simulink model "generic_20231123_1032"  (R2022b)
settings: Solver=ode45  StartTime=0.0  StopTime=50  RelTol=1e-3  EnableMultiTasking=on
model workspace (MAT data in the model file):
  A = 1
  B = 1.19071237887
  kd = -9.99955278144
  ki = 0.00519416981022
  kp = 9.99999979837
undefined symbols (not defined in the file): brake_select, curvature, DiscIntNeverNeededParam, speed
libraries: CarMaker4SL x88, simulink x1, mpcadaslib x1
(part 2 of 4)

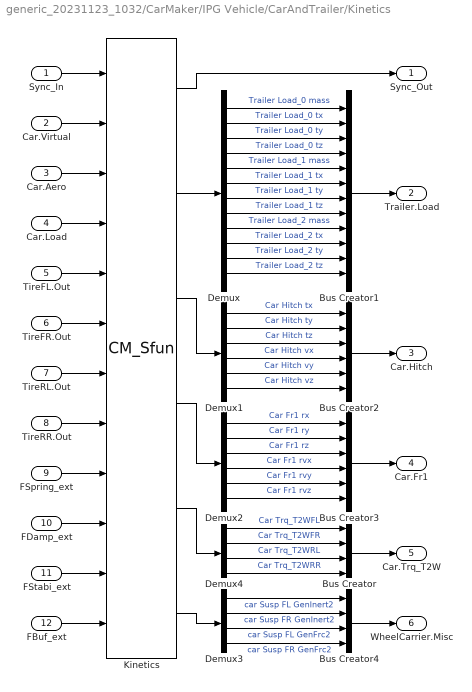
== system generic_20231123_1032/CarMaker/IPG Vehicle/CarAndTrailer/Kinetics ==
  Sync_In : Inport
  Car.Virtual : Inport  Port=2
  Car.Aero : Inport  Port=3
  Car.Load : Inport  Port=4
  TireFL.Out : Inport  Port=5
  TireFR.Out : Inport  Port=6
  TireRL.Out : Inport  Port=7
  TireRR.Out : Inport  Port=8
  FSpring_ext : Inport  Port=9
  FDamp_ext : Inport  Port=10
  FStabi_ext : Inport  Port=11
  FBuf_ext : Inport  Port=12
  Bus Creator : BusCreator  Inputs=4
  Bus Creator1 : BusCreator  Inputs=12
  Bus Creator2 : BusCreator  Inputs=6
  Bus Creator3 : BusCreator  Inputs=6
  Bus Creator4 : BusCreator  Inputs=4
  Demux : Demux  Outputs=12
      settings: DisplayOption=none
  Demux1 : Demux  Outputs=6
      settings: DisplayOption=none
  Demux2 : Demux  Outputs=6
      settings: DisplayOption=none
  Demux3 : Demux
      settings: DisplayOption=none
  Demux4 : Demux
      settings: DisplayOption=none
  Kinetics : S-Function  FunctionName=CM_Sfun  Parameters='Kinetics'  SFunctionDeploymentMode=off  EnableBusSupport=off
  Sync_Out : Outport  VectorParamsAs1DForOutWhenUnconnected=off
  Trailer.Load : Outport  Port=2  VectorParamsAs1DForOutWhenUnconnected=off
  Car.Hitch : Outport  Port=3  VectorParamsAs1DForOutWhenUnconnected=off
  Car.Fr1 : Outport  Port=4  VectorParamsAs1DForOutWhenUnconnected=off
  Car.Trq_T2W : Outport  Port=5  VectorParamsAs1DForOutWhenUnconnected=off
  WheelCarrier.Misc : Outport  Port=6  VectorParamsAs1DForOutWhenUnconnected=off
  wires:
  FBuf_ext/1 -> Kinetics/12
  Sync_In/1 -> Kinetics/1
  Kinetics/1 -> Sync_Out/1
  Car.Aero/1 -> Kinetics/3
  Car.Virtual/1 -> Kinetics/2
  Bus Creator1/1 -> Trailer.Load/1
  Demux/1 -> Bus Creator1/1  "Trailer Load_0 mass"
  Demux/2 -> Bus Creator1/2  "Trailer Load_0 tx"
  Demux/3 -> Bus Creator1/3  "Trailer Load_0 ty"
  Demux/4 -> Bus Creator1/4  "Trailer Load_0 tz"
  Kinetics/2 -> Demux/1
  Demux/5 -> Bus Creator1/5  "Trailer Load_1 mass"
  Demux/6 -> Bus Creator1/6  "Trailer Load_1 tx"
  Demux/7 -> Bus Creator1/7  "Trailer Load_1 ty"
  Demux/8 -> Bus Creator1/8  "Trailer Load_1 tz"
  Demux/9 -> Bus Creator1/9  "Trailer Load_2 mass"
  Demux/10 -> Bus Creator1/10  "Trailer Load_2 tx"
  Demux/11 -> Bus Creator1/11  "Trailer Load_2 ty"
  Demux/12 -> Bus Creator1/12  "Trailer Load_2 tz"
  Demux1/1 -> Bus Creator2/1  "Car Hitch tx"
  Demux1/2 -> Bus Creator2/2  "Car Hitch ty"
  Demux1/3 -> Bus Creator2/3  "Car Hitch tz"
  Demux1/4 -> Bus Creator2/4  "Car Hitch vx"
  Demux1/5 -> Bus Creator2/5  "Car Hitch vy"
  Demux1/6 -> Bus Creator2/6  "Car Hitch vz"
  Kinetics/3 -> Demux1/1
  Bus Creator2/1 -> Car.Hitch/1
  Demux2/1 -> Bus Creator3/1  "Car Fr1 rx"
  Demux2/2 -> Bus Creator3/2  "Car Fr1 ry"
  Demux2/3 -> Bus Creator3/3  "Car Fr1 rz"
  Demux2/4 -> Bus Creator3/4  "Car Fr1 rvx"
  Demux2/5 -> Bus Creator3/5  "Car Fr1 rvy"
  Demux2/6 -> Bus Creator3/6  "Car Fr1 rvz"
  Bus Creator3/1 -> Car.Fr1/1
  Kinetics/4 -> Demux2/1
  Car.Load/1 -> Kinetics/4
  Demux3/1 -> Bus Creator4/1  "car Susp FL GenInert2"
  Demux3/2 -> Bus Creator4/2  "car Susp FR GenInert2"
  Demux3/3 -> Bus Creator4/3  "car Susp FL GenFrc2"
  Demux3/4 -> Bus Creator4/4  "car Susp FR GenFrc2"
  Bus Creator4/1 -> WheelCarrier.Misc/1
  Bus Creator/1 -> Car.Trq_T2W/1
  Demux4/4 -> Bus Creator/4  "Car Trq_T2WRR"
  Demux4/3 -> Bus Creator/3  "Car Trq_T2WRL"
  Demux4/2 -> Bus Creator/2  "Car Trq_T2WFR"
  Demux4/1 -> Bus Creator/1  "Car Trq_T2WFL"
  TireFL.Out/1 -> Kinetics/5
  TireFR.Out/1 -> Kinetics/6
  TireRL.Out/1 -> Kinetics/7
  TireRR.Out/1 -> Kinetics/8
  FSpring_ext/1 -> Kinetics/9
  FDamp_ext/1 -> Kinetics/10
  FStabi_ext/1 -> Kinetics/11
  Kinetics/6 -> Demux3/1
  Kinetics/5 -> Demux4/1

== system generic_20231123_1032/CarMaker/IPG Vehicle/CarAndTrailer/Steering ==
  note: When replacing the entire steering system,
      | be sure to disable the IPG steering model by using the steering
      | model 'Model Manager off' in the vehicle GUI.
  Sync_In : Inport
  VhclCtrl.Steering : Inport  Port=2
  Bus Creator1 : BusCreator  Inputs=16
  Bus Creator2 : BusCreator  Inputs=5
  Demux : Demux  Outputs=21
      settings: DisplayOption=none
  Steering : S-Function  FunctionName=CM_Sfun  Parameters='Steering'  SFunctionDeploymentMode=off  EnableBusSupport=off
  Terminator : Terminator
  Sync_Out : Outport  VectorParamsAs1DForOutWhenUnconnected=off
  Steer.IF : Outport  Port=2  VectorParamsAs1DForOutWhenUnconnected=off
  wires:
  Demux/21 -> Bus Creator2/5  "Steering IF R Inert"
  Demux/20 -> Bus Creator2/4  "Steering IF R Frc"
  Demux/19 -> Bus Creator2/3  "Steering IF L Inert"
  Demux/18 -> Bus Creator2/2  "Steering IF L Frc"
  Demux/17 -> Bus Creator2/1  "Steering IF SteerByTrq"
  Demux/16 -> Bus Creator1/16  "Steering IF R iSteer2q"
  Demux/15 -> Bus Creator1/15  "Steering IF R qpp"
  Demux/14 -> Bus Creator1/14  "Steering IF R qp"
  Demux/13 -> Bus Creator1/13  "Steering IF R q"
  Demux/12 -> Bus Creator1/12  "Steering IF L iSteer2q"
  Demux/11 -> Bus Creator1/11  "Steering IF L qpp"
  Demux/10 -> Bus Creator1/10  "Steering IF L qp"
  Demux/9 -> Bus Creator1/9  "Steering IF L q"
  Demux/8 -> Bus Creator1/8  "Steering IF AssistTrqPin"
  Demux/7 -> Bus Creator1/7  "Steering IF AssistTrqCol"
  Demux/6 -> Bus Creator1/6  "Steering IF AssistFrc"
  Demux/5 -> Bus Creator1/5  "Steering IF TrqStatic"
  Demux/4 -> Bus Creator1/4  "Steering IF Trq"
  Demux/3 -> Bus Creator1/3  "Steering IF AngAcc"
  Demux/2 -> Bus Creator1/2  "Steering IF AngVel"
  Demux/1 -> Bus Creator1/1  "Steering IF Ang"
  Bus Creator1/1 -> Steer.IF/1
  Steering/2 -> Demux/1
  Bus Creator2/1 -> Terminator/1  "Steer IF (in)"
  VhclCtrl.Steering/1 -> Steering/2
  Steering/1 -> Sync_Out/1
  Sync_In/1 -> Steering/1

== system generic_20231123_1032/CarMaker/IPG Vehicle/CarAndTrailer/Trailer ==
  Sync_In : Inport
  Trailer.Load : Inport  Port=2
  Car.Hitch : Inport  Port=3
  Car.Fr1 : Inport  Port=4
  Car.Trq_T2W : Inport  Port=5
  WheelCarrier.Misc : Inport  Port=6
  CreateBus Car.Hitch.FrcTrq : Subsystem
  CreateBus Vhcl.Motion : Subsystem
  CreateBus Vhcl.PoI : Subsystem
  CreateBus Vhcl.Steering : Subsystem
  CreateBus Vhcl.Wheel.FL : Subsystem
  CreateBus Vhcl.Wheel.FR : Subsystem
  CreateBus Vhcl.Wheel.RL : Subsystem
  CreateBus Vhcl.Wheel.RR : Subsystem
  Trailer : S-Function  FunctionName=CM_Sfun  Parameters='Trailer'  SFunctionDeploymentMode=off  EnableBusSupport=off
  Sync_Out : Outport  VectorParamsAs1DForOutWhenUnconnected=off
  Vhcl.Steering : Outport  Port=2  VectorParamsAs1DForOutWhenUnconnected=off
  Vhcl.Motion : Outport  Port=3  VectorParamsAs1DForOutWhenUnconnected=off
  Vhcl.PoI : Outport  Port=4  VectorParamsAs1DForOutWhenUnconnected=off
  Vhcl.Wheel.FL : Outport  Port=5  VectorParamsAs1DForOutWhenUnconnected=off
  Vhcl.Wheel.FR : Outport  Port=6  VectorParamsAs1DForOutWhenUnconnected=off
  Vhcl.Wheel.RL : Outport  Port=7  VectorParamsAs1DForOutWhenUnconnected=off
  Vhcl.Wheel.RR : Outport  Port=8  VectorParamsAs1DForOutWhenUnconnected=off
  Car.Hitch.FrcTrq : Outport  Port=9  VectorParamsAs1DForOutWhenUnconnected=off
  wires:
  Trailer/2 -> CreateBus Vhcl.Steering/1(In1)
  CreateBus Vhcl.Steering/1(Out1) -> Vhcl.Steering/1  "Vhcl.Steering"
  Trailer/3 -> CreateBus Vhcl.Motion/1(In1)
  Trailer/4 -> CreateBus Vhcl.PoI/1(In1)
  Trailer/5 -> CreateBus Vhcl.Wheel.FL/1(In1)
  Trailer/6 -> CreateBus Vhcl.Wheel.FR/1(In1)
  Trailer/7 -> CreateBus Vhcl.Wheel.RL/1(In1)
  Trailer/9 -> CreateBus Car.Hitch.FrcTrq/1(In1)
  Trailer/8 -> CreateBus Vhcl.Wheel.RR/1(In1)
  CreateBus Vhcl.Wheel.RR/1(Out1) -> Vhcl.Wheel.RR/1  "Vhcl.Wheel.RR"
  CreateBus Vhcl.Wheel.RL/1(Out1) -> Vhcl.Wheel.RL/1  "Vhcl.Wheel.RL"
  CreateBus Vhcl.Wheel.FR/1(Out1) -> Vhcl.Wheel.FR/1  "Vhcl.Wheel.FR"
  CreateBus Vhcl.Wheel.FL/1(Out1) -> Vhcl.Wheel.FL/1  "Vhcl.Wheel.FL"
  CreateBus Vhcl.PoI/1(Out1) -> Vhcl.PoI/1  "Vhcl.PoI"
  CreateBus Vhcl.Motion/1(Out1) -> Vhcl.Motion/1  "Vhcl.Motion"
  Car.Trq_T2W/1 -> Trailer/5
  WheelCarrier.Misc/1 -> Trailer/6
  CreateBus Car.Hitch.FrcTrq/1(Out1) -> Car.Hitch.FrcTrq/1  "Car.Hitch.FrcTrq"
  Car.Fr1/1 -> Trailer/4
  Car.Hitch/1 -> Trailer/3
  Trailer.Load/1 -> Trailer/2
  Trailer/1 -> Sync_Out/1
  Sync_In/1 -> Trailer/1

== system generic_20231123_1032/CarMaker/VehicleControl/CreateBus VhclCtrl/A*algoithm ==
  Bus Selector1 : BusSelector  OutputSignals=Path.tx,Path.ty
  Constant : Constant  Value=0
  Constant3 : Constant  Value=0
  Constant4 : Constant
  Gain : Gain  Gain=2
  MATLAB Function1 : MATLAB Function  TreatAsAtomicUnit=on
  Mux : Mux  Inputs=2
  Mux1 : Mux  Inputs=2
  Mux2 : Mux  Inputs=2
  Read CM Dict3 : CarMaker4SL/Read CM Dict  xname=Sensor.Radar.VehSensor_6.Obj0.Length  xsync=off  xstime=Continuous
  Read CM Dict4 : CarMaker4SL/Read CM Dict  xname=Traffic.T00.tx  xsync=off  xstime=Continuous
  Read CM Dict5 : CarMaker4SL/Read CM Dict  xname=Traffic.T00.ty  xsync=off  xstime=Continuous
  Read CM Dict6 : CarMaker4SL/Read CM Dict  xname=Sensor.Radar.VehSensor_6.Obj0.ProbObst  xsync=off  xstime=Continuous
  Read CM Dict7 : CarMaker4SL/Read CM Dict  xname=Sensor.Radar.VehSensor_6.Obj0.Width  xsync=off  xstime=Continuous
  Reshape : Reshape  OutputDimensionality=Customize  OutputDimensions=[1,2]
  Reshape1 : Reshape  OutputDimensionality=Customize  OutputDimensions=[1,2]
  Reshape2 : Reshape  OutputDimensionality=Customize  OutputDimensions=[1,2]
  Road Sensor1 : CarMaker4SL/Sensors/Road Sensor  xname=0  xstime=Continuous
      settings: SourceProductName=CarMaker4SL
  Sum : Sum  Inputs=|++
  Switch : Switch  Criteria=u2 > Threshold  SaturateOnIntegerOverflow=off  InputSameDT=off
  Out1 : Outport
  deviation : Outport  Port=2
  pathX : Outport  Port=3
  pathY : Outport  Port=4
  wires:
  Read CM Dict3/1 -> Gain/1
  Read CM Dict4/1 -> Mux1/1, Mux/1
  Read CM Dict5/1 -> Sum/2, Mux/2
  Read CM Dict7/1 -> ?
  Constant3/1 -> Road Sensor1/1
  Bus Selector1/1 -> Mux2/1  "<tx>"
  Constant/1 -> Switch/3
  Road Sensor1/1 -> Out1/1
  Constant4/1 -> Switch/1
  Switch/1 -> ?
  Read CM Dict6/1 -> Switch/2
  Bus Selector1/2 -> Mux2/2  "<ty>"
  Road Sensor1/2 -> Bus Selector1/1
  MATLAB Function1/3(pathY) -> pathY/1
  MATLAB Function1/1(deviation) -> deviation/1
  MATLAB Function1/2(pathX) -> pathX/1
  Mux2/1 -> Reshape/1
  Mux/1 -> Reshape2/1
  Sum/1 -> Mux1/2
  Gain/1 -> Sum/1
  Mux1/1 -> Reshape1/1
  Reshape/1 -> MATLAB Function1/1(start)
  Reshape1/1 -> MATLAB Function1/2(target)
  Reshape2/1 -> MATLAB Function1/3(obstacles)

== system generic_20231123_1032/CarMaker/VehicleControl/CreateBus VhclCtrl/Stanley_controller ==
  Path Out : Inport
  Yaw_re : Inport  Port=2
  Abs : Abs  SaturateOnIntegerOverflow=off
  Abs1 : Abs  SaturateOnIntegerOverflow=off
  Constant : Constant
  Constant1 : Constant
  Constant2 : Constant  Value=30/3.6
  Constant3 : Constant  Value=A
  Constant4 : Constant  Value=B
  Display : Display
  Gain1 : Gain  Gain=3.6
  Gain2 : Gain  Gain=3.6
  MATLAB Function : MATLAB Function  TreatAsAtomicUnit=on
  Memory3 : Memory
  Memory4 : Memory
  Read CM Dict : CarMaker4SL/Read CM Dict  xname=Vhcl.v  xsync=off  xstime=Continuous
  Scope : Scope  NumInputPorts=2
  Stanley : Subsystem  Commented=on
  Throttle : Outport
  Target_Steering_angle_rad : Outport  Port=2
  Brake_command : Outport  Port=3
  wires:
  Stanley/3(Brake_command) -> Brake_command/1
  Stanley/1(Target_Steering_angle_rad) -> Target_Steering_angle_rad/1
  [Yaw_m] -> Stanley/4(<Yaw_angle_rad>)
  Memory3/1 -> Stanley/3(<Vy_Global_m_s>)
  Memory4/1 -> Stanley/2(<Vx_Global_m_s>)
  Path Out/1 -> Stanley/1(Path_out)
  Constant1/1 -> Abs1/1
  Constant2/1 -> MATLAB Function/1(speed_rf), Stanley/6(Desired_speed), Gain2/1
  Constant/1 -> Abs/1
  Yaw_re/1 -> [Yaw_m]
  Abs/1 -> Display/1, Memory4/1
  Abs1/1 -> Memory3/1
  Read CM Dict/1 -> MATLAB Function/2(current_speed), Gain1/1, Stanley/5(<Actual_Velocity_Car_m_s>)
  Constant3/1 -> MATLAB Function/3(A)
  Constant4/1 -> MATLAB Function/4(B)
  Gain1/1 -> Scope/1
  Stanley/2(Throttle) -> Throttle/1
  Gain2/1 -> Scope/2

== system generic_20231123_1032/CarMaker/VehicleControl/CreateBus VhclCtrl/Subsystem ==
  Bus Selector : BusSelector  OutputSignals=Route.tx,Route.ty
  Constant : Constant  Value=0
  Constant1 : Constant  Value=0
  Read CM Dict : CarMaker4SL/Read CM Dict  xname=Sensor.Radar.VehSensor_6.Obj0.DistX  xsync=off  xstime=Continuous
  Read CM Dict1 : CarMaker4SL/Read CM Dict  xname=Sensor.Radar.VehSensor_6.Obj0.DistY  xsync=off  xstime=Continuous
  Read CM Dict3 : CarMaker4SL/Read CM Dict  xname=Sensor.Radar.VehSensor_6.Obj0.ProbObst  xsync=off  xstime=Continuous
  Road Sensor : CarMaker4SL/Sensors/Road Sensor  xname=0  xstime=Continuous
      settings: SourceProductName=CarMaker4SL
  Sum : Sum  Inputs=|++
  Sum1 : Sum  Inputs=|++
  Switch : Switch  Criteria=u2 > Threshold  SaturateOnIntegerOverflow=off  InputSameDT=off
  Switch1 : Switch  Criteria=u2 > Threshold  SaturateOnIntegerOverflow=off  InputSameDT=off
  Out1 : Outport
  Out2 : Outport  Port=2
  Out3 : Outport  Port=3
  wires:
  Read CM Dict1/1 -> Sum/1
  Sum/1 -> Switch/1
  Constant/1 -> Switch1/3, Switch/3
  Sum1/1 -> Switch1/1
  Switch/1 -> Out1/1
  Bus Selector/2 -> Sum1/1  "<ty>"
  Read CM Dict3/1 -> Switch1/2, Switch/2
  Read CM Dict/1 -> Sum1/2
  Road Sensor/2 -> Bus Selector/1
  Constant1/1 -> Road Sensor/1
  Bus Selector/1 -> Sum/2  "<tx>"
  Road Sensor/1 -> Out3/1
  Switch1/1 -> Out2/1

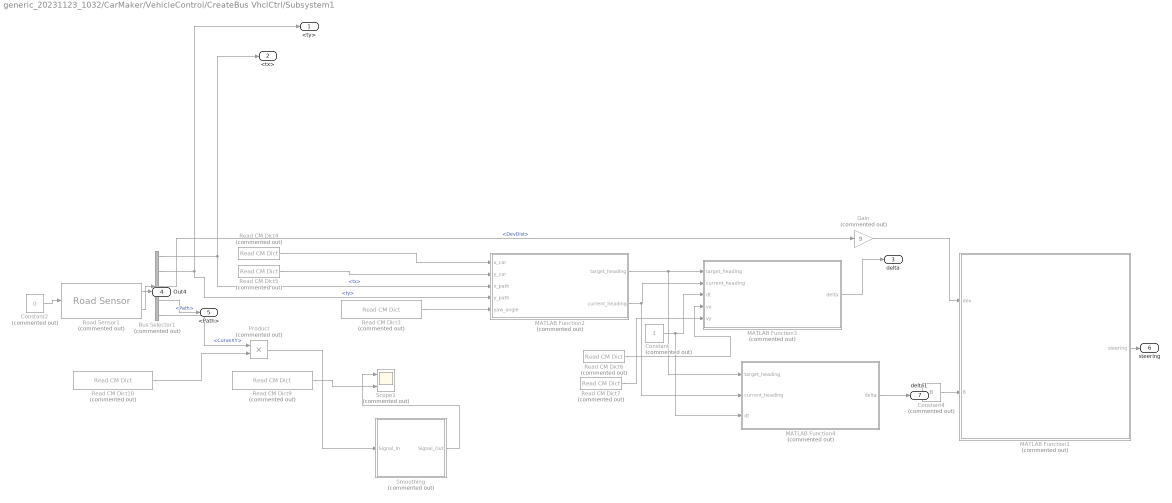
== system generic_20231123_1032/CarMaker/VehicleControl/CreateBus VhclCtrl/Subsystem1 ==
  Bus Selector1 : BusSelector  Commented=on  OutputSignals=Path.tx,Path.ty,Path.DevDist,Path,Path.CurveXY
  Constant : Constant  Commented=on
  Constant2 : Constant  Commented=on  Value=0
  Constant4 : Constant  Commented=on  Value=B
  Gain : Gain  Commented=on  Gain=9
  MATLAB Function1 : MATLAB Function  Commented=on  TreatAsAtomicUnit=on
  MATLAB Function2 : MATLAB Function  Commented=on  TreatAsAtomicUnit=on
  MATLAB Function3 : MATLAB Function  Commented=on  TreatAsAtomicUnit=on
  MATLAB Function4 : MATLAB Function  Commented=on  TreatAsAtomicUnit=on
  Product : Product  Commented=on
  Read CM Dict10 : CarMaker4SL/Read CM Dict  Commented=on  xname=Vhcl.v  xsync=off  xstime=Continuous
  Read CM Dict3 : CarMaker4SL/Read CM Dict  Commented=on  xname=Vhcl.Yaw  xsync=off  xstime=Continuous
  Read CM Dict4 : CarMaker4SL/Read CM Dict  Commented=on  xname=Car.Con.tx  xsync=off  xstime=Continuous
  Read CM Dict5 : CarMaker4SL/Read CM Dict  Commented=on  xname=Car.Con.ty  xsync=off  xstime=Continuous
  Read CM Dict6 : CarMaker4SL/Read CM Dict  Commented=on  xname=Car.Con.vx_1  xsync=off  xstime=Continuous
  Read CM Dict7 : CarMaker4SL/Read CM Dict  Commented=on  xname=Car.Con.vy_1  xsync=off  xstime=Continuous
  Read CM Dict9 : CarMaker4SL/Read CM Dict  Commented=on  xname=Car.YawRate  xsync=off  xstime=Continuous
  Road Sensor1 : CarMaker4SL/Sensors/Road Sensor  Commented=on  xname=0  xstime=Continuous
      settings: SourceProductName=CarMaker4SL
  Scope1 : Scope  Commented=on  NumInputPorts=2
  Smoothing : Subsystem  Commented=on
  <ty> : Outport
  <tx> : Outport  Port=2
  delta : Outport  Port=3
  Out4 : Outport  Port=4
  <Path> : Outport  Port=5
  steering : Outport  Port=6
  delta1 : Outport  Port=7
  wires:
  MATLAB Function2/2(current_heading) -> MATLAB Function4/2(current_heading), MATLAB Function3/2(current_heading)
  MATLAB Function2/1(target_heading) -> MATLAB Function4/1(target_heading), MATLAB Function3/1(target_heading)
  Read CM Dict3/1 -> MATLAB Function2/5(yaw_angle)
  Bus Selector1/2 -> <ty>/1, MATLAB Function2/4(y_path)  "<ty>"
  Read CM Dict7/1 -> MATLAB Function3/5(vy)
  Constant/1 -> MATLAB Function4/3(dt), MATLAB Function3/3(dt)
  Read CM Dict5/1 -> MATLAB Function2/2(y_car)
  Road Sensor1/2 -> Bus Selector1/1
  Read CM Dict6/1 -> MATLAB Function3/4(vx)
  Read CM Dict10/1 -> Product/2
  MATLAB Function1/1(steering) -> steering/1
  Bus Selector1/3 -> Gain/1  "<DevDist>"
  MATLAB Function3/1(delta) -> delta/1
  Smoothing/1(Signal_Out) -> Scope1/1
  Product/1 -> Smoothing/1(Signal_In)
  Bus Selector1/1 -> <tx>/1, MATLAB Function2/3(x_path)  "<tx>"
  Gain/1 -> MATLAB Function1/1(dev)
  Constant4/1 -> MATLAB Function1/2(B)
  Read CM Dict4/1 -> MATLAB Function2/1(x_car)
  Read CM Dict9/1 -> Scope1/2
  Bus Selector1/5 -> Product/1  "<CurveXY>"
  Constant2/1 -> Road Sensor1/1
  Bus Selector1/4 -> <Path>/1  "<Path>"
  MATLAB Function4/1(delta) -> delta1/1
  Road Sensor1/1 -> Out4/1

== system generic_20231123_1032/CarMaker/VehicleControl/CreateBus VhclCtrl/Subsystem2 ==
  In1 : Inport
  Bus Selector2 : BusSelector  Commented=on  OutputSignals=Path.tx,Path.ty,Path.DevDist,Path.CurveXY,Path
  Constant3 : Constant  Commented=on  Value=0
  Delay2 : Delay  Commented=on  DelayLength=1
  Delay3 : Delay  Commented=on  DelayLength=1
  MATLAB Function7 : MATLAB Function  Commented=on  TreatAsAtomicUnit=on
  Read CM Dict14 : CarMaker4SL/Read CM Dict  Commented=on  xname=Car.Gen.ty  xsync=off  xstime=Continuous
  Read CM Dict15 : CarMaker4SL/Read CM Dict  Commented=on  xname=Car.Gen.tx  xsync=off  xstime=Continuous
  Road Sensor2 : CarMaker4SL/Sensors/Road Sensor  Commented=on  xname=0  xstime=Continuous
      settings: SourceProductName=CarMaker4SL
  Sum : Sum  Commented=on  Inputs=|++
  Sum1 : Sum  Commented=on  Inputs=|++
  Out1 : Outport
  cte : Outport  Port=2
  <DevDist> : Outport  Port=3
  <CurveXY> : Outport  Port=4
  denominator : Outport  Port=5
  <Path> : Outport  Port=6
  wires:
  Bus Selector2/2 -> Delay2/1, MATLAB Function7/4(y_point)  "<ty>"
  Road Sensor2/2 -> Bus Selector2/1
  In1/1 -> Sum/2, Sum1/2
  Read CM Dict15/1 -> MATLAB Function7/1(x_vehicle)
  Sum/1 -> MATLAB Function7/3(x_point)
  Delay3/1 -> Sum1/1
  Sum1/1 -> MATLAB Function7/5(x2)
  Bus Selector2/1 -> Delay3/1, Sum/1  "<tx>"
  Delay2/1 -> MATLAB Function7/6(y2)
  Constant3/1 -> Road Sensor2/1
  Read CM Dict14/1 -> MATLAB Function7/2(y_vehicle)
  Bus Selector2/3 -> <DevDist>/1  "<DevDist>"
  MATLAB Function7/1(cte) -> cte/1
  Bus Selector2/4 -> <CurveXY>/1  "<CurveXY>"
  MATLAB Function7/2(denominator) -> denominator/1
  Road Sensor2/1 -> Out1/1
  Bus Selector2/5 -> <Path>/1  "<Path>"

== system generic_20231123_1032/CarMaker/VehicleControl/CreateBus VhclCtrl/Subsystem3 ==
  In1 : Inport
  y2 : Inport  Port=2
  x2 : Inport  Port=3
  Delay : Delay  Commented=on  DelayLength=1
  Delay1 : Delay  Commented=on  DelayLength=1
  Gain1 : Gain  Commented=on  Gain=-1
  MATLAB Function5 : MATLAB Function  Commented=on  TreatAsAtomicUnit=on
  Read CM Dict12 : CarMaker4SL/Read CM Dict  Commented=on  xname=Car.Gen.ty  xsync=off  xstime=Continuous
  Read CM Dict8 : CarMaker4SL/Read CM Dict  Commented=on  xname=Car.Gen.tx  xsync=off  xstime=Continuous
  Sign : Signum  Commented=on
  Out1 : Outport
  denominator : Outport  Port=2
  Out3 : Outport  Port=3
  wires:
  y2/1 -> Delay/1, MATLAB Function5/6(y2)
  x2/1 -> Delay1/1, MATLAB Function5/5(x2)
  Read CM Dict8/1 -> MATLAB Function5/1(x_vehicle)
  Delay/1 -> MATLAB Function5/4(y_point)
  Sign/1 -> Out3/1
  Read CM Dict12/1 -> MATLAB Function5/2(y_vehicle)
  Delay1/1 -> MATLAB Function5/3(x_point)
  MATLAB Function5/1(cte) -> Gain1/1
  MATLAB Function5/2(denominator) -> denominator/1
  Gain1/1 -> Out1/1
  In1/1 -> Sign/1

== system generic_20231123_1032/CarMaker/VehicleControl/CreateBus VhclCtrl/Subsystem4 ==
  y_dev : Inport
  Constant5 : Constant  Value=1.97
  Gain2 : Gain  Gain=-1
  MATLAB Function6 : MATLAB Function  TreatAsAtomicUnit=on
  MATLAB Function8 : MATLAB Function  Commented=on  TreatAsAtomicUnit=on
  Read CM Dict : CarMaker4SL/Read CM Dict  xname=Sensor.Object.VehSensor_5.relvTgt.NearPnt.ds.y  xsync=off  xstime=Continuous
  Read CM Dict1 : CarMaker4SL/Read CM Dict  xname=Car.Road.Path.DevDist  xsync=off  xstime=Continuous
  Read CM Dict11 : CarMaker4SL/Read CM Dict  xname=Sensor.Object.RadarL.relvTgt.NearPnt.ds.y  xsync=off  xstime=Continuous
  Read CM Dict13 : CarMaker4SL/Read CM Dict  xname=Sensor.Object.RadarL.Obj.T00.RefPnt.ds.x  xsync=off  xstime=Continuous
  Read CM Dict16 : CarMaker4SL/Read CM Dict  xname=Sensor.Object.VehSensor_4.relvTgt.NearPnt.ds.y  xsync=off  xstime=Continuous
  Read CM Dict17 : CarMaker4SL/Read CM Dict  xname=Sensor.Object.RadarL.relvTgt.NearPnt.ds.x  xsync=off  xstime=Continuous
  Scope : Scope  NumInputPorts=2
  Subsystem : Subsystem
  y_added : Outport
  Signal_In : Outport  Port=2
  wires:
  Read CM Dict/1 -> MATLAB Function6/5(y_error), MATLAB Function8/2(data)
  MATLAB Function6/1(error) -> Gain2/1, Scope/2
  Read CM Dict11/1 -> MATLAB Function6/4(y_error_2)
  Read CM Dict13/1 -> MATLAB Function8/3(distance), Scope/1, MATLAB Function6/6(distance)
  Gain2/1 -> Subsystem/1(In1)
  Read CM Dict1/1 -> MATLAB Function6/1(path_dev)
  Read CM Dict16/1 -> MATLAB Function6/3(y_error3)
  Constant5/1 -> MATLAB Function6/2(y_dev)
  Read CM Dict17/1 -> MATLAB Function6/7(x_distance_obj)
  Subsystem/1(Signal_In) -> Signal_In/1
  y_dev/1 -> MATLAB Function8/1(y_dev)
  MATLAB Function8/1(y_added) -> y_added/1

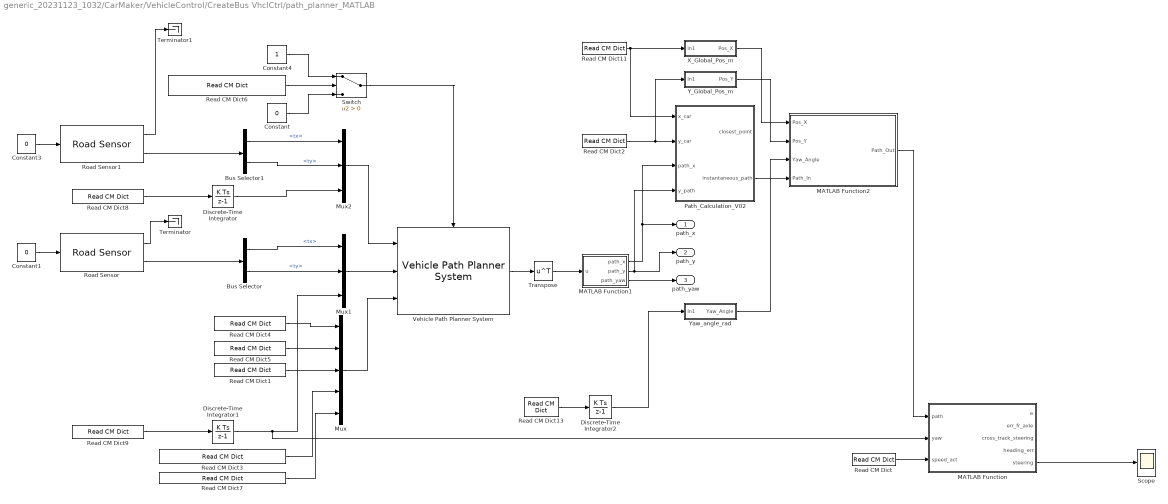
== system generic_20231123_1032/CarMaker/VehicleControl/CreateBus VhclCtrl/path_planner_MATLAB ==
  Bus Selector : BusSelector  OutputSignals=Path.tx,Path.ty
  Bus Selector1 : BusSelector  OutputSignals=Path.tx,Path.ty
  Constant : Constant  Value=0
  Constant1 : Constant  Value=0
  Constant3 : Constant  Value=0
  Constant4 : Constant
  Discrete-Time Integrator : DiscreteIntegrator  SampleTime=-1  ICPrevOutput=DiscIntNeverNeededParam  ICPrevScaledInput=DiscIntNeverNeededParam
  Discrete-Time Integrator1 : DiscreteIntegrator  SampleTime=-1  ICPrevOutput=DiscIntNeverNeededParam  ICPrevScaledInput=DiscIntNeverNeededParam
  Discrete-Time Integrator2 : DiscreteIntegrator  SampleTime=-1  ICPrevOutput=DiscIntNeverNeededParam  ICPrevScaledInput=DiscIntNeverNeededParam
  MATLAB Function : MATLAB Function  TreatAsAtomicUnit=on
  MATLAB Function1 : MATLAB Function  TreatAsAtomicUnit=on
  MATLAB Function2 : MATLAB Function  TreatAsAtomicUnit=on
  Mux : Mux  Inputs=5
  Mux1 : Mux  Inputs=3
  Mux2 : Mux  Inputs=3
  Path_Calculation_V02 : MATLAB Function  TreatAsAtomicUnit=on
  Read CM Dict : CarMaker4SL/Read CM Dict  xname=Vhcl.v  xsync=off  xstime=Continuous
  Read CM Dict1 : CarMaker4SL/Read CM Dict  xname=Traffic.T00.rz  xsync=off  xstime=Continuous
  Read CM Dict11 : CarMaker4SL/Read CM Dict  xname=Car.Gen.tx  xsync=off  xstime=Continuous
  Read CM Dict13 : CarMaker4SL/Read CM Dict  xname=Car.YawRate  xsync=off  xstime=Continuous
  Read CM Dict2 : CarMaker4SL/Read CM Dict  xname=Car.Gen.ty  xsync=off  xstime=Continuous
  Read CM Dict3 : CarMaker4SL/Read CM Dict  xname=Sensor.Radar.VehSensor_6.Obj0.Length  xsync=off  xstime=Continuous
  Read CM Dict4 : CarMaker4SL/Read CM Dict  xname=Traffic.T00.tx  xsync=off  xstime=Continuous
  Read CM Dict5 : CarMaker4SL/Read CM Dict  xname=Traffic.T00.ty  xsync=off  xstime=Continuous
  Read CM Dict6 : CarMaker4SL/Read CM Dict  xname=Sensor.Radar.VehSensor_6.Obj0.ProbObst  xsync=off  xstime=Continuous
  Read CM Dict7 : CarMaker4SL/Read CM Dict  xname=Sensor.Radar.VehSensor_6.Obj0.Width  xsync=off  xstime=Continuous
  Read CM Dict8 : CarMaker4SL/Read CM Dict  xname=Car.YawRate  xsync=off  xstime=Continuous
  Read CM Dict9 : CarMaker4SL/Read CM Dict  xname=Car.YawRate  xsync=off  xstime=Continuous
  Road Sensor : CarMaker4SL/Sensors/Road Sensor  xname=0  xstime=Continuous
      settings: SourceProductName=CarMaker4SL
  Road Sensor1 : CarMaker4SL/Sensors/Road Sensor  xname=0  xstime=Continuous
      settings: SourceProductName=CarMaker4SL
  Scope : Scope
  Switch : Switch  Criteria=u2 > Threshold  SaturateOnIntegerOverflow=off  InputSameDT=off
  Terminator : Terminator
  Terminator1 : Terminator
  Transpose : Math  Operator=transpose
  Vehicle Path Planner System : mpcadaslib/Vehicle Path Planner System  egoLength=4.7  egoWidth=1.8  wheelbase=2.8  dist2Center=1.4  numObs=1  obsMat=zeros(1,5)  obs_ext=on  minDist=1  Ts=1  pPlanning=20  v_range=[-20,30]  v_ext=off  steer_range=[-pi/4,pi/4]  steer_ext=off  suboptimal=off  maxiter=200  output_exitflag=off
      settings: LibrarySourceBlock=mpclib/Automated Driving/Vehicle Path Planner System
  X_Global_Pos_m : Subsystem
  Y_Global_Pos_m : Subsystem
  Yaw_angle_rad : Subsystem
  path_x : Outport
  path_y : Outport  Port=2
  path_yaw : Outport  Port=3
  wires:
  Constant3/1 -> Road Sensor1/1
  Road Sensor/1 -> Terminator/1
  Read CM Dict8/1 -> Discrete-Time Integrator/1
  Constant1/1 -> Road Sensor/1
  Mux2/1 -> Vehicle Path Planner System/1
  Road Sensor1/1 -> Terminator1/1
  Road Sensor1/2 -> Bus Selector1/1
  Road Sensor/2 -> Bus Selector/1
  MATLAB Function1/2(path_y) -> path_y/1, Path_Calculation_V02/4(y_path)
  Read CM Dict9/1 -> Discrete-Time Integrator1/1
  Constant4/1 -> Switch/1
  Read CM Dict6/1 -> Switch/2
  Discrete-Time Integrator1/1 -> MATLAB Function/2(yaw), Mux1/3
  Constant/1 -> Switch/3
  Bus Selector1/2 -> Mux2/2  "<ty>"
  Bus Selector1/1 -> Mux2/1  "<tx>"
  Yaw_angle_rad/1(Yaw_Angle) -> MATLAB Function2/3(Yaw_Angle)
  Y_Global_Pos_m/1(Pos_Y) -> MATLAB Function2/2(Pos_Y)
  Discrete-Time Integrator/1 -> Mux2/3
  Read CM Dict/1 -> MATLAB Function/3(speed_act)
  Bus Selector/1 -> Mux1/1  "<tx>"
  Bus Selector/2 -> Mux1/2  "<ty>"
  Read CM Dict4/1 -> Mux/1
  Read CM Dict5/1 -> Mux/2
  X_Global_Pos_m/1(Pos_X) -> MATLAB Function2/1(Pos_X)
  Discrete-Time Integrator2/1 -> Yaw_angle_rad/1(In1)
  Read CM Dict2/1 -> Path_Calculation_V02/2(y_car), Y_Global_Pos_m/1(In1)
  Read CM Dict11/1 -> Path_Calculation_V02/1(x_car), X_Global_Pos_m/1(In1)
  Read CM Dict1/1 -> Mux/3
  Read CM Dict3/1 -> Mux/4
  Read CM Dict7/1 -> Mux/5
  Switch/1 -> Vehicle Path Planner System/Enable
  Transpose/1 -> MATLAB Function1/1(u)
  Vehicle Path Planner System/1 -> Transpose/1
  Mux1/1 -> Vehicle Path Planner System/2
  Mux/1 -> Vehicle Path Planner System/3
  MATLAB Function2/1(Path_Out) -> MATLAB Function/1(path)
  Read CM Dict13/1 -> Discrete-Time Integrator2/1
  MATLAB Function1/1(path_x) -> Path_Calculation_V02/3(path_x), path_x/1
  MATLAB Function1/3(path_yaw) -> path_yaw/1
  Path_Calculation_V02/2(instantaneous_path) -> MATLAB Function2/4(Path_In)
  MATLAB Function/5(steering) -> Scope/1

== system generic_20231123_1032/CarMaker/VehicleControl/Stanley controller/Crosstrack_steering ==
  speed : Inport
  Abs : Abs  SaturateOnIntegerOverflow=off
  Atan : Trigonometry  Operator=atan
  Constant : Constant  Value=6
  Constant1 : Constant
  Divide : Product  Inputs=*/
  Gain : Gain  Gain=-1
  Product : Product
  Read CM Dict5 : CarMaker4SL/Read CM Dict  xname=Car.Road.Path.DevDist  xsync=off  xstime=Continuous
  Sum1 : Sum  Inputs=|++
  Out1 : Outport
  wires:
  Atan/1 -> Out1/1
  Divide/1 -> Atan/1
  Constant1/1 -> Sum1/1
  speed/1 -> Sum1/2
  Constant/1 -> Product/2
  Sum1/1 -> Divide/2
  Product/1 -> Gain/1
  Read CM Dict5/1 -> Abs/1
  Abs/1 -> Product/1
  Gain/1 -> Divide/1

== system generic_20231123_1032/CarMaker/VehicleControl/Stanley controller/Stanley controller version_1 ==
  Direction : Inport
  Stanley controller version_1 : Subsystem  VariantControl=Choice  ReferencedSubsystem=Stanley_controller_version_1
  Radians out : Outport
  SteerCmd : Outport  Port=2

== system generic_20231123_1032/CarMaker/VehicleControl/Stanley controller/Steady_state_yaw ==
  V : Inport
  Curvature : Inport  Port=2
  Constant : Constant  Value=1600.00
  Constant1 : Constant  Value=70551.0
  Constant3 : Constant  Value=1.488
  Constant4 : Constant  Value=1.487
  Constant5 : Constant  Value=1.5
  Divide : Product  Inputs=*/
  Divide1 : Product  Inputs=*/
  Product : Product  Inputs=3
  Product1 : Product
  Square : Math  Operator=square
  Sum : Sum  Inputs=|++
  Steady_state_yaw : Outport
  wires:
  Constant5/1 -> Sum/1
  Constant4/1 -> Divide/1
  Constant3/1 -> Divide/2
  V/1 -> Square/1
  Constant/1 -> Product/2
  Divide/1 -> Sum/2
  Sum/1 -> Product1/2
  Square/1 -> Product/1
  Curvature/1 -> Product/3
  Product/1 -> Divide1/1
  Constant1/1 -> Product1/1
  Product1/1 -> Divide1/2
  Divide1/1 -> Steady_state_yaw/1

== system generic_20231123_1032/CarMaker/VehicleControl/Stanley controller/Subsystem ==
  In1 : Inport
  Add : Sum  Inputs=+++
  Derivative : Derivative
  Discrete-Time Integrator : DiscreteIntegrator  SampleTime=-1  ICPrevOutput=DiscIntNeverNeededParam  ICPrevScaledInput=DiscIntNeverNeededParam
  Gain : Gain  Gain=0.6
  Gain1 : Gain  Gain=1.2
  Gain2 : Gain  Gain=0.4
  Signal_In : Outport
  wires:
  Gain1/1 -> Discrete-Time Integrator/1
  Gain2/1 -> Derivative/1
  Discrete-Time Integrator/1 -> Add/1
  Derivative/1 -> Add/3
  Gain/1 -> Add/2
  In1/1 -> Gain/1, Gain2/1, Gain1/1
  Add/1 -> Signal_In/1

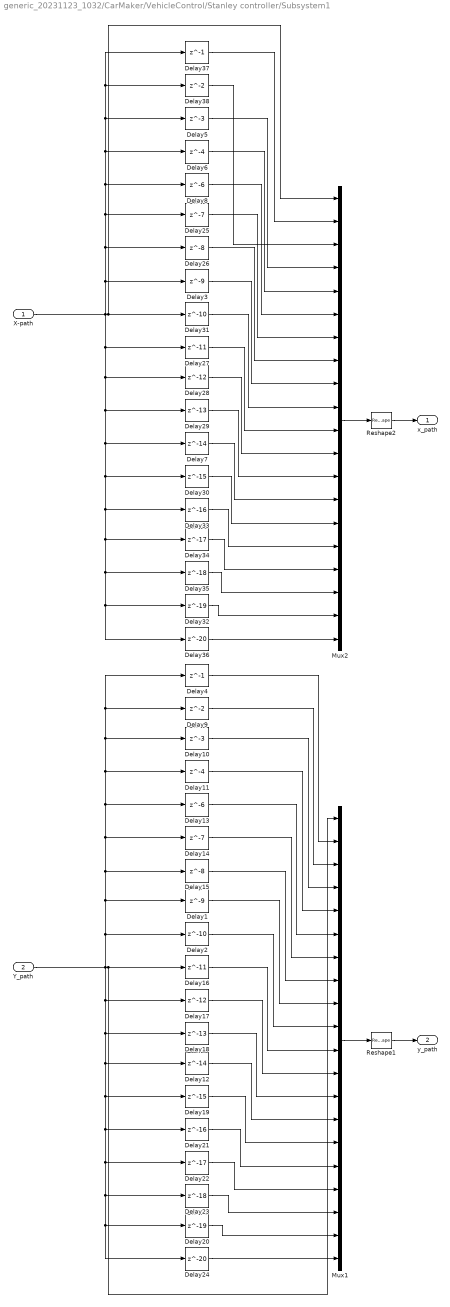
== system generic_20231123_1032/CarMaker/VehicleControl/Stanley controller/Subsystem1 ==
  X-path : Inport
  Y_path : Inport  Port=2
  Delay1 : Delay  DelayLength=9
  Delay10 : Delay  DelayLength=3
  Delay11 : Delay  DelayLength=4
  Delay12 : Delay  DelayLength=14
  Delay13 : Delay  DelayLength=6
  Delay14 : Delay  DelayLength=7
  Delay15 : Delay  DelayLength=8
  Delay16 : Delay  DelayLength=11
  Delay17 : Delay  DelayLength=12
  Delay18 : Delay  DelayLength=13
  Delay19 : Delay  DelayLength=15
  Delay2 : Delay  DelayLength=10
  Delay20 : Delay  DelayLength=19
  Delay21 : Delay  DelayLength=16
  Delay22 : Delay  DelayLength=17
  Delay23 : Delay  DelayLength=18
  Delay24 : Delay  DelayLength=20
  Delay25 : Delay  DelayLength=7
  Delay26 : Delay  DelayLength=8
  Delay27 : Delay  DelayLength=11
  Delay28 : Delay  DelayLength=12
  Delay29 : Delay  DelayLength=13
  Delay3 : Delay  DelayLength=9
  Delay30 : Delay  DelayLength=15
  Delay31 : Delay  DelayLength=10
  Delay32 : Delay  DelayLength=19
  Delay33 : Delay  DelayLength=16
  Delay34 : Delay  DelayLength=17
  Delay35 : Delay  DelayLength=18
  Delay36 : Delay  DelayLength=20
  Delay37 : Delay  DelayLength=1
  Delay38 : Delay
  Delay4 : Delay  DelayLength=1
  Delay5 : Delay  DelayLength=3
  Delay6 : Delay  DelayLength=4
  Delay7 : Delay  DelayLength=14
  Delay8 : Delay  DelayLength=6
  Delay9 : Delay
  Mux1 : Mux  Inputs=20
  Mux2 : Mux  Inputs=20
  Reshape1 : Reshape  OutputDimensionality=Customize  OutputDimensions=[1,20]
  Reshape2 : Reshape  OutputDimensionality=Customize  OutputDimensions=[1,20]
  x_path : Outport
  y_path : Outport  Port=2
  wires:
  Delay12/1 -> Mux1/14
  X-path/1 -> Delay32/1, Delay36/1, Delay35/1, Delay34/1, Delay33/1, Delay30/1, Delay7/1, Delay29/1, Delay28/1, Delay27/1, Delay31/1, Mux2/1, Delay38/1, Delay37/1, Delay5/1, Delay6/1, Delay8/1, Delay25/1, Delay26/1, Delay3/1
  Delay25/1 -> Mux2/7
  Delay17/1 -> Mux1/12
  Y_path/1 -> Delay20/1, Delay24/1, Delay23/1, Delay22/1, Delay21/1, Delay19/1, Delay12/1, Delay18/1, Delay17/1, Mux1/1, Delay16/1, Delay4/1, Delay9/1, Delay10/1, Delay11/1, Delay13/1, Delay14/1, Delay15/1, Delay1/1, Delay2/1
  Delay5/1 -> Mux2/4
  Delay37/1 -> Mux2/2
  Delay6/1 -> Mux2/5
  Delay38/1 -> Mux2/3
  Delay20/1 -> Mux1/19
  Delay18/1 -> Mux1/13
  Delay8/1 -> Mux2/6
  Delay26/1 -> Mux2/8
  Delay3/1 -> Mux2/9
  Delay31/1 -> Mux2/10
  Delay27/1 -> Mux2/11
  Delay24/1 -> Mux1/20
  Delay28/1 -> Mux2/12
  Delay29/1 -> Mux2/13
  Delay7/1 -> Mux2/14
  Delay30/1 -> Mux2/15
  Delay33/1 -> Mux2/16
  Mux1/1 -> Reshape1/1
  Delay34/1 -> Mux2/17
  Delay35/1 -> Mux2/18
  Delay1/1 -> Mux1/9
  Delay32/1 -> Mux2/19
  Delay15/1 -> Mux1/8
  Delay36/1 -> Mux2/20
  Reshape1/1 -> y_path/1
  Delay4/1 -> Mux1/2
  Delay16/1 -> Mux1/11
  Delay9/1 -> Mux1/3
  Delay21/1 -> Mux1/16
  Delay10/1 -> Mux1/4
  Delay11/1 -> Mux1/5
  Delay13/1 -> Mux1/6
  Reshape2/1 -> x_path/1
  Delay14/1 -> Mux1/7
  Delay2/1 -> Mux1/10
  Delay19/1 -> Mux1/15
  Delay22/1 -> Mux1/17
  Delay23/1 -> Mux1/18
  Mux2/1 -> Reshape2/1

== system generic_20231123_1032/CarMaker/VehicleControl/Stanley controller/Subsystem3 ==
  X-path : Inport
  Y_path : Inport  Port=2
  Delay37 : Delay  DelayLength=1
  Delay4 : Delay  DelayLength=1
  Mux1 : Mux  Inputs=2
  Mux2 : Mux  Inputs=2
  Reshape1 : Reshape  OutputDimensionality=Customize  OutputDimensions=[1,2]
  Reshape2 : Reshape  OutputDimensionality=Customize  OutputDimensions=[1,2]
  x_path : Outport
  y_path : Outport  Port=2
  wires:
  X-path/1 -> Delay37/1, Mux2/1
  Y_path/1 -> Delay4/1, Mux1/1
  Delay37/1 -> Mux2/2
  Mux1/1 -> Reshape1/1
  Reshape1/1 -> y_path/1
  Delay4/1 -> Mux1/2
  Reshape2/1 -> x_path/1
  Mux2/1 -> Reshape2/1

== system generic_20231123_1032/CarMaker/VehicleControl/Stanley controller/X_Global_Pos_m ==
  In1 : Inport
  Pos_X : Outport  VectorParamsAs1DForOutWhenUnconnected=off
  wires:
  In1/1 -> Pos_X/1

== system generic_20231123_1032/CarMaker/VehicleControl/Stanley controller/Y_Global_Pos_m ==
  In1 : Inport
  Pos_Y : Outport  VectorParamsAs1DForOutWhenUnconnected=off
  wires:
  In1/1 -> Pos_Y/1

== system generic_20231123_1032/CarMaker/VehicleControl/Stanley controller/Yaw_angle_rad ==
  In1 : Inport
  Yaw_Angle : Outport  VectorParamsAs1DForOutWhenUnconnected=off
  wires:
  In1/1 -> Yaw_Angle/1

== system generic_20231123_1032/CarMaker/IPG Vehicle/CarAndTrailer/CarAndTrailerUpd/CreateBus Brake.IF.In ==
  In : Inport
  BusCreator : BusCreator  Inputs=9
  Demux : Demux  Outputs=9
      settings: DisplayOption=none
  Out : Outport  VectorParamsAs1DForOutWhenUnconnected=off
  wires:
  Demux/9 -> BusCreator/9  "Brake IF Trq_Reg RR"
  Demux/8 -> BusCreator/8  "Brake IF Trq_Reg RL"
  Demux/7 -> BusCreator/7  "Brake IF Trq_Reg FR"
  Demux/6 -> BusCreator/6  "Brake IF Trq_Reg FL"
  Demux/5 -> BusCreator/5  "Brake IF Trq_Reg_max RR"
  Demux/4 -> BusCreator/4  "Brake IF Trq_Reg_max RL"
  Demux/3 -> BusCreator/3  "Brake IF Trq_Reg_max FR"
  Demux/2 -> BusCreator/2  "Brake IF Trq_Reg_max FL"
  Demux/1 -> BusCreator/1  "Brake IF T_env"
  BusCreator/1 -> Out/1
  In/1 -> Demux/1

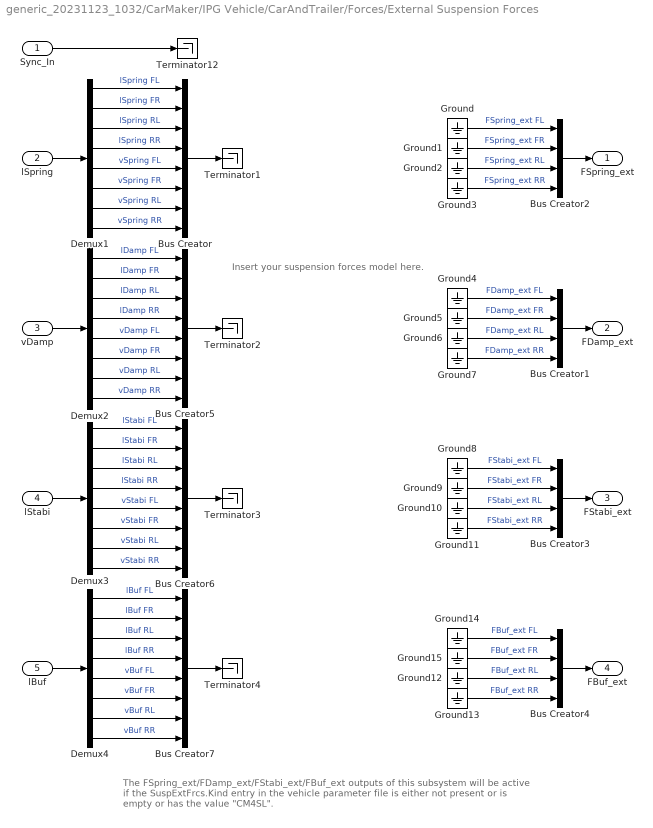
== system generic_20231123_1032/CarMaker/IPG Vehicle/CarAndTrailer/Forces/External Suspension Forces ==
  note: The FSpring_ext/FDamp_ext/FStabi_ext/FBuf_ext outputs of this subsystem will be
      | active if the SuspExtFrcs.Kind entry in the vehicle parameter file
      | is either not present or is empty or has the value "CM4SL".
  note: Insert your suspension forces model here.
  Sync_In : Inport
  lSpring : Inport  Port=2
  vDamp : Inport  Port=3
  lStabi : Inport  Port=4
  lBuf : Inport  Port=5
  Bus Creator{,5..7} (4 alike) : BusCreator  Inputs=8
  Bus Creator{1..4} (4 alike) : BusCreator  Inputs=4
  Demux{1..4} (4 alike) : Demux  Outputs=8
      settings: DisplayOption=none
  Ground{,1..15} (16 alike) : Ground
  Terminator{1..4,12} (5 alike) : Terminator
  FSpring_ext : Outport  VectorParamsAs1DForOutWhenUnconnected=off
  FDamp_ext : Outport  Port=2  VectorParamsAs1DForOutWhenUnconnected=off
  FStabi_ext : Outport  Port=3  VectorParamsAs1DForOutWhenUnconnected=off
  FBuf_ext : Outport  Port=4  VectorParamsAs1DForOutWhenUnconnected=off
  wires:
  Bus Creator7/1 -> Terminator4/1
  Bus Creator6/1 -> Terminator3/1
  Bus Creator5/1 -> Terminator2/1
  Bus Creator/1 -> Terminator1/1
  Demux4/8 -> Bus Creator7/8  "vBuf RR"
  Demux4/7 -> Bus Creator7/7  "vBuf RL"
  Demux4/6 -> Bus Creator7/6  "vBuf FR"
  Demux4/5 -> Bus Creator7/5  "vBuf FL"
  Demux3/8 -> Bus Creator6/8  "vStabi RR"
  Demux3/7 -> Bus Creator6/7  "vStabi RL"
  Demux3/6 -> Bus Creator6/6  "vStabi FR"
  Demux3/5 -> Bus Creator6/5  "vStabi FL"
  Demux2/8 -> Bus Creator5/8  "vDamp RR"
  Demux2/7 -> Bus Creator5/7  "vDamp RL"
  Demux2/6 -> Bus Creator5/6  "vDamp FR"
  Demux2/5 -> Bus Creator5/5  "vDamp FL"
  Demux1/8 -> Bus Creator/8  "vSpring RR"
  Demux1/7 -> Bus Creator/7  "vSpring RL"
  Demux1/6 -> Bus Creator/6  "vSpring FR"
  Demux1/5 -> Bus Creator/5  "vSpring FL"
  Demux2/4 -> Bus Creator5/4  "lDamp RR"
  Demux2/3 -> Bus Creator5/3  "lDamp RL"
  Demux2/2 -> Bus Creator5/2  "lDamp FR"
  Demux2/1 -> Bus Creator5/1  "lDamp FL"
  Demux1/4 -> Bus Creator/4  "lSpring RR"
  Demux1/3 -> Bus Creator/3  "lSpring RL"
  Demux1/2 -> Bus Creator/2  "lSpring FR"
  Demux1/1 -> Bus Creator/1  "lSpring FL"
  Demux3/4 -> Bus Creator6/4  "lStabi RR"
  Demux3/3 -> Bus Creator6/3  "lStabi RL"
  Demux3/2 -> Bus Creator6/2  "lStabi FR"
  Demux3/1 -> Bus Creator6/1  "lStabi FL"
  lStabi/1 -> Demux3/1
  vDamp/1 -> Demux2/1
  lSpring/1 -> Demux1/1
  Demux4/4 -> Bus Creator7/4  "lBuf RR"
  Demux4/3 -> Bus Creator7/3  "lBuf RL"
  Demux4/2 -> Bus Creator7/2  "lBuf FR"
  Demux4/1 -> Bus Creator7/1  "lBuf FL"
  lBuf/1 -> Demux4/1
  Ground14/1 -> Bus Creator4/1  "FBuf_ext FL"
  Ground15/1 -> Bus Creator4/2  "FBuf_ext FR"
  Ground12/1 -> Bus Creator4/3  "FBuf_ext RL"
  Ground13/1 -> Bus Creator4/4  "FBuf_ext RR"
  Bus Creator4/1 -> FBuf_ext/1
  Sync_In/1 -> Terminator12/1
  Bus Creator2/1 -> FSpring_ext/1
  Ground/1 -> Bus Creator2/1  "FSpring_ext FL"
  Ground1/1 -> Bus Creator2/2  "FSpring_ext FR"
  Ground2/1 -> Bus Creator2/3  "FSpring_ext RL"
  Ground3/1 -> Bus Creator2/4  "FSpring_ext RR"
  Ground4/1 -> Bus Creator1/1  "FDamp_ext FL"
  Ground5/1 -> Bus Creator1/2  "FDamp_ext FR"
  Ground6/1 -> Bus Creator1/3  "FDamp_ext RL"
  Ground7/1 -> Bus Creator1/4  "FDamp_ext RR"
  Bus Creator1/1 -> FDamp_ext/1
  Ground8/1 -> Bus Creator3/1  "FStabi_ext FL"
  Ground9/1 -> Bus Creator3/2  "FStabi_ext FR"
  Ground10/1 -> Bus Creator3/3  "FStabi_ext RL"
  Ground11/1 -> Bus Creator3/4  "FStabi_ext RR"
  Bus Creator3/1 -> FStabi_ext/1

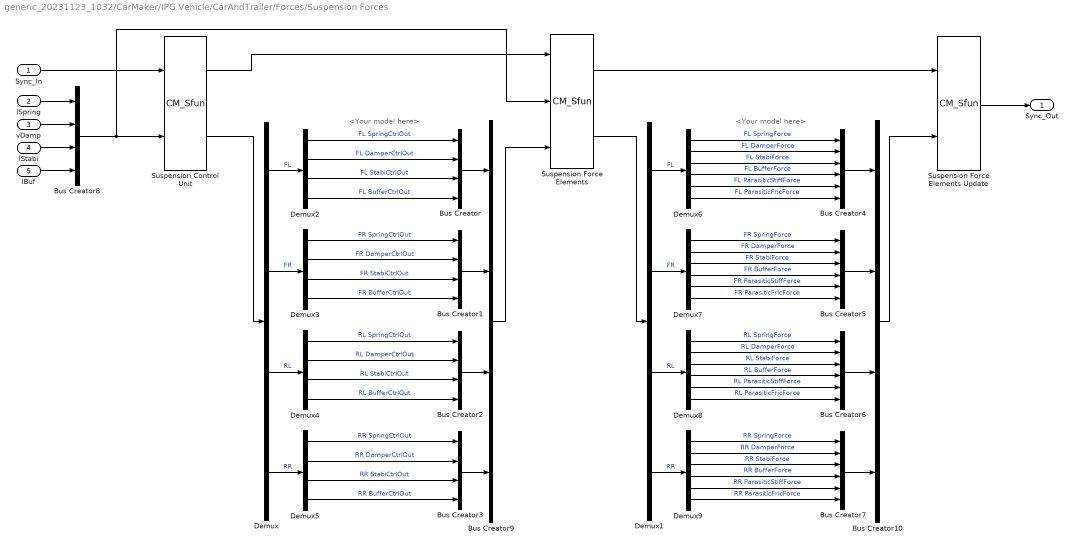
== system generic_20231123_1032/CarMaker/IPG Vehicle/CarAndTrailer/Forces/Suspension Forces ==
  note: <Your model here>
  note: <Your model here>
  Sync_In : Inport
  lSpring : Inport  Port=2
  vDamp : Inport  Port=3
  lStabi : Inport  Port=4
  lBuf : Inport  Port=5
  Bus Creator{,1..3,8..10} (7 alike) : BusCreator  Inputs=4
  Bus Creator{4..7} (4 alike) : BusCreator  Inputs=6
  Demux{,1..5} (6 alike) : Demux
  Demux{6..9} (4 alike) : Demux  Outputs=6
  Suspension Control Unit : S-Function  FunctionName=CM_Sfun  Parameters='ForcesSuspControl'  SFunctionDeploymentMode=off  EnableBusSupport=off
  Suspension Force Elements : S-Function  FunctionName=CM_Sfun  Parameters='ForcesSusp'  SFunctionDeploymentMode=off  EnableBusSupport=off
  Suspension Force Elements Update : S-Function  FunctionName=CM_Sfun  Parameters='ForcesSuspUpd'  SFunctionDeploymentMode=off  EnableBusSupport=off
  Sync_Out : Outport  VectorParamsAs1DForOutWhenUnconnected=off
  wires:
  vDamp/1 -> Bus Creator8/2
  lStabi/1 -> Bus Creator8/3
  lBuf/1 -> Bus Creator8/4
  lSpring/1 -> Bus Creator8/1
  Bus Creator8/1 -> Suspension Control Unit/2, Suspension Force Elements/2
  Sync_In/1 -> Suspension Control Unit/1
  Suspension Control Unit/1 -> Suspension Force Elements/1
  Suspension Force Elements/1 -> Suspension Force Elements Update/1
  Suspension Force Elements Update/1 -> Sync_Out/1
  Bus Creator4/1 -> Bus Creator10/1
  Bus Creator5/1 -> Bus Creator10/2
  Bus Creator6/1 -> Bus Creator10/3
  Bus Creator7/1 -> Bus Creator10/4
  Demux6/1 -> Bus Creator4/1  "FL SpringForce"
  Demux9/1 -> Bus Creator7/1  "RR SpringForce"
  Demux9/2 -> Bus Creator7/2  "RR DamperForce"
  Demux9/3 -> Bus Creator7/3  "RR StabiForce"
  Demux9/4 -> Bus Creator7/4  "RR BufferForce"
  Demux9/5 -> Bus Creator7/5  "RR ParasiticStiffForce"
  Demux9/6 -> Bus Creator7/6  "RR ParasiticFricForce"
  Demux8/1 -> Bus Creator6/1  "RL SpringForce"
  Demux8/2 -> Bus Creator6/2  "RL DamperForce"
  Demux8/4 -> Bus Creator6/4  "RL BufferForce"
  Demux8/5 -> Bus Creator6/5  "RL ParasiticStiffForce"
  Demux8/6 -> Bus Creator6/6  "RL ParasiticFricForce"
  Demux8/3 -> Bus Creator6/3  "RL StabiForce"
  Demux7/1 -> Bus Creator5/1  "FR SpringForce"
  Demux7/2 -> Bus Creator5/2  "FR DamperForce"
  Demux7/3 -> Bus Creator5/3  "FR StabiForce"
  Demux7/4 -> Bus Creator5/4  "FR BufferForce"
  Demux7/5 -> Bus Creator5/5  "FR ParasiticStiffForce"
  Demux7/6 -> Bus Creator5/6  "FR ParasiticFricForce"
  Demux6/2 -> Bus Creator4/2  "FL DamperForce"
  Demux6/3 -> Bus Creator4/3  "FL StabiForce"
  Demux6/4 -> Bus Creator4/4  "FL BufferForce"
  Demux6/5 -> Bus Creator4/5  "FL ParasiticStiffForce"
  Demux6/6 -> Bus Creator4/6  "FL ParasiticFricForce"
  Bus Creator10/1 -> Suspension Force Elements Update/2
  Demux/1 -> Demux2/1  "FL"
  Bus Creator1/1 -> Bus Creator9/2
  Demux/2 -> Demux3/1  "FR"
  Bus Creator2/1 -> Bus Creator9/3
  Demux/3 -> Demux4/1  "RL"
  Bus Creator3/1 -> Bus Creator9/4
  Demux2/1 -> Bus Creator/1  "FL SpringCtrlOut"
  Demux/4 -> Demux5/1  "RR"
  Demux5/1 -> Bus Creator3/1  "RR SpringCtrlOut"
  Demux5/2 -> Bus Creator3/2  "RR DamperCtrlOut"
  Demux5/3 -> Bus Creator3/3  "RR StabiCtrlOut"
  Demux5/4 -> Bus Creator3/4  "RR BufferCtrlOut"
  Demux4/1 -> Bus Creator2/1  "RL SpringCtrlOut"
  Demux4/2 -> Bus Creator2/2  "RL DamperCtrlOut"
  Demux4/4 -> Bus Creator2/4  "RL BufferCtrlOut"
  Demux4/3 -> Bus Creator2/3  "RL StabiCtrlOut"
  Demux3/1 -> Bus Creator1/1  "FR SpringCtrlOut"
  Demux3/2 -> Bus Creator1/2  "FR DamperCtrlOut"
  Demux3/3 -> Bus Creator1/3  "FR StabiCtrlOut"
  Demux3/4 -> Bus Creator1/4  "FR BufferCtrlOut"
  Demux2/2 -> Bus Creator/2  "FL DamperCtrlOut"
  Demux2/3 -> Bus Creator/3  "FL StabiCtrlOut"
  Demux2/4 -> Bus Creator/4  "FL BufferCtrlOut"
  Suspension Control Unit/2 -> Demux/1
  Bus Creator9/1 -> Suspension Force Elements/3
  Bus Creator/1 -> Bus Creator9/1
  Suspension Force Elements/2 -> Demux1/1
  Demux1/1 -> Demux6/1  "FL"
  Demux1/2 -> Demux7/1  "FR"
  Demux1/3 -> Demux8/1  "RL"
  Demux1/4 -> Demux9/1  "RR"

== system generic_20231123_1032/CarMaker/IPG Vehicle/CarAndTrailer/Forces/Tires ==
  note: The TireXX_Out signals will only be used if FileIdent is "CarMaker-Tire-CM4SL" in the tire parameter file!
      | An example parameter file can be found in Data/Tire/DT_CM4SL_UserTire.
  Sync_In : Inport
  TireFL_In : Inport  Port=2
  TireFR_In : Inport  Port=3
  TireRL_In : Inport  Port=4
  TireRR_In : Inport  Port=5
  Bus Creator{1..4} (4 alike) : BusCreator  Inputs=11
  Demux{1..3,8} (4 alike) : Demux  Outputs=7
      settings: DisplayOption=none
  TireFL : Subsystem
  TireFR : Subsystem
  TireRL : Subsystem
  TireRR : Subsystem
  TireFL_Out : Outport  VectorParamsAs1DForOutWhenUnconnected=off
  TireFR_Out : Outport  Port=2  VectorParamsAs1DForOutWhenUnconnected=off
  TireRL_Out : Outport  Port=3  VectorParamsAs1DForOutWhenUnconnected=off
  TireRR_Out : Outport  Port=4  VectorParamsAs1DForOutWhenUnconnected=off
  wires:
  Sync_In/1 -> TireRR/1(Sync_In), TireRL/1(Sync_In), TireFR/1(Sync_In), TireFL/1(Sync_In)
  Bus Creator4/1 -> TireRR_Out/1
  Bus Creator2/1 -> TireRL_Out/1
  Bus Creator1/1 -> TireFR_Out/1
  Demux3/5 -> TireRR/6(Rim_turnv)  "Tire_In Rim_turnv"
  Demux3/4 -> TireRR/5(Rim_rotv)  "Tire_In Rim_rotv"
  Demux3/1 -> TireRR/2(Load)  "Tire_In Load"
  Demux3/7 -> TireRR/8(muRoad)  "Tire_In mu"
  Demux3/6 -> TireRR/7(InclinAngle)  "Tire_In Camber"
  Demux3/2 -> TireRR/3(vxtrans)  "Tire_In vxtrans"
  Demux3/3 -> TireRR/4(vytrans)  "Tire_In vytrans"
  TireRR/11(AlignTrq) -> Bus Creator4/11  "Tire_Out AlignTrq"
  TireRR/10(RollResist) -> Bus Creator4/10  "Tire_Out RollResist"
  TireRR/9(OverturnTrq) -> Bus Creator4/9  "Tire_Out OverturnTrq"
  TireRR/8(LoadFrc) -> Bus Creator4/8  "Tire_Out LoadFrc"
  TireRR/7(SideFrc) -> Bus Creator4/7  "Tire_Out SideFrc"
  TireRR/6(LongFrc) -> Bus Creator4/6  "Tire_Out LongFrc"
  TireRR/5(vBelt) -> Bus Creator4/5  "Tire_Out vBelt"
  TireRR/4(rBelt_eff) -> Bus Creator4/4  "Tire_Out rBelt_eff"
  TireRR/3(TurnSlp) -> Bus Creator4/3  "Tire_Out TurnSlp"
  TireRR/1(Slp) -> Bus Creator4/1  "Tire_Out Slp"
  TireRR/2(Alpha) -> Bus Creator4/2  "Tire_Out Alpha"
  Demux2/5 -> TireRL/6(Rim_turnv)  "Tire_In Rim_turnv"
  Demux2/4 -> TireRL/5(Rim_rotv)  "Tire_In Rim_rotv"
  Demux2/1 -> TireRL/2(Load)  "Tire_In Load"
  Demux2/7 -> TireRL/8(muRoad)  "Tire_In mu"
  Demux2/6 -> TireRL/7(InclinAngle)  "Tire_In Camber"
  Demux2/2 -> TireRL/3(vxtrans)  "Tire_In vxtrans"
  Demux2/3 -> TireRL/4(vytrans)  "Tire_In vytrans"
  TireRL/11(AlignTrq) -> Bus Creator2/11  "Tire_Out AlignTrq"
  TireRL/10(RollResist) -> Bus Creator2/10  "Tire_Out RollResist"
  TireRL/9(OverturnTrq) -> Bus Creator2/9  "Tire_Out OverturnTrq"
  TireRL/8(LoadFrc) -> Bus Creator2/8  "Tire_Out LoadFrc"
  TireRL/7(SideFrc) -> Bus Creator2/7  "Tire_Out SideFrc"
  TireRL/6(LongFrc) -> Bus Creator2/6  "Tire_Out LongFrc"
  TireRL/5(vBelt) -> Bus Creator2/5  "Tire_Out vBelt"
  TireRL/4(rBelt_eff) -> Bus Creator2/4  "Tire_Out rBelt_eff"
  TireRL/3(TurnSlp) -> Bus Creator2/3  "Tire_Out TurnSlp"
  TireRL/1(Slp) -> Bus Creator2/1  "Tire_Out Slp"
  TireRL/2(Alpha) -> Bus Creator2/2  "Tire_Out Alpha"
  Demux1/5 -> TireFR/6(Rim_turnv)  "Tire_In Rim_turnv"
  Demux1/4 -> TireFR/5(Rim_rotv)  "Tire_In Rim_rotv"
  Demux1/1 -> TireFR/2(Load)  "Tire_In Load"
  Demux1/7 -> TireFR/8(muRoad)  "Tire_In mu"
  Demux1/6 -> TireFR/7(InclinAngle)  "Tire_In Camber"
  Demux1/2 -> TireFR/3(vxtrans)  "Tire_In vxtrans"
  Demux1/3 -> TireFR/4(vytrans)  "Tire_In vytrans"
  TireFR/11(AlignTrq) -> Bus Creator1/11  "Tire_Out AlignTrq"
  TireFR/10(RollResist) -> Bus Creator1/10  "Tire_Out RollResist"
  TireFR/9(OverturnTrq) -> Bus Creator1/9  "Tire_Out OverturnTrq"
  TireFR/8(LoadFrc) -> Bus Creator1/8  "Tire_Out LoadFrc"
  TireFR/7(SideFrc) -> Bus Creator1/7  "Tire_Out SideFrc"
  TireFR/6(LongFrc) -> Bus Creator1/6  "Tire_Out LongFrc"
  TireFR/5(vBelt) -> Bus Creator1/5  "Tire_Out vBelt"
  TireFR/4(rBelt_eff) -> Bus Creator1/4  "Tire_Out rBelt_eff"
  TireFR/3(TurnSlp) -> Bus Creator1/3  "Tire_Out TurnSlp"
  TireFR/1(Slp) -> Bus Creator1/1  "Tire_Out Slp"
  TireFR/2(Alpha) -> Bus Creator1/2  "Tire_Out Alpha"
  Demux8/5 -> TireFL/6(Rim_turnv)  "Tire_In Rim_turnv"
  Demux8/4 -> TireFL/5(Rim_rotv)  "Tire_In Rim_rotv"
  TireFL_In/1 -> Demux8/1
  Demux8/1 -> TireFL/2(Load)  "Tire_In Load"
  Demux8/7 -> TireFL/8(muRoad)  "Tire_In mu"
  Demux8/6 -> TireFL/7(InclinAngle)  "Tire_In Camber"
  Demux8/2 -> TireFL/3(vxtrans)  "Tire_In vxtrans"
  Demux8/3 -> TireFL/4(vytrans)  "Tire_In vytrans"
  TireFL/11(AlignTrq) -> Bus Creator3/11  "Tire_Out AlignTrq"
  TireFL/10(RollResist) -> Bus Creator3/10  "Tire_Out RollResist"
  TireFL/9(OverturnTrq) -> Bus Creator3/9  "Tire_Out OverturnTrq"
  TireFL/8(LoadFrc) -> Bus Creator3/8  "Tire_Out LoadFrc"
  TireFL/7(SideFrc) -> Bus Creator3/7  "Tire_Out SideFrc"
  TireFL/6(LongFrc) -> Bus Creator3/6  "Tire_Out LongFrc"
  TireFL/5(vBelt) -> Bus Creator3/5  "Tire_Out vBelt"
  TireFL/4(rBelt_eff) -> Bus Creator3/4  "Tire_Out rBelt_eff"
  TireFL/3(TurnSlp) -> Bus Creator3/3  "Tire_Out TurnSlp"
  TireFL/1(Slp) -> Bus Creator3/1  "Tire_Out Slp"
  TireFL/2(Alpha) -> Bus Creator3/2  "Tire_Out Alpha"
  Bus Creator3/1 -> TireFL_Out/1
  TireFR_In/1 -> Demux1/1
  TireRL_In/1 -> Demux2/1
  TireRR_In/1 -> Demux3/1

== system generic_20231123_1032/CarMaker/IPG Vehicle/CarAndTrailer/Forces/Vehicle Forces ==
  Sync_In : Inport
  Bus Creator1 : BusCreator  Inputs=12
  Bus Creator8 : BusCreator  Inputs=16
  BusCreator1 : BusCreator  Inputs=4
  BusCreator2 : BusCreator  Inputs=9
  Demux : Demux  Outputs=16
      settings: DisplayOption=none
  Demux1 : Demux  Outputs=12
      settings: DisplayOption=none
  Demux2 : Demux  Outputs=13
      settings: DisplayOption=none
  Forces : S-Function  FunctionName=CM_Sfun  Parameters='Forces'  SFunctionDeploymentMode=off  EnableBusSupport=off
  Terminator : Terminator
  Sync_Out : Outport  VectorParamsAs1DForOutWhenUnconnected=off
  Car.Virtual : Outport  Port=2  VectorParamsAs1DForOutWhenUnconnected=off
  Car.Aero : Outport  Port=3  VectorParamsAs1DForOutWhenUnconnected=off
  Car.Load : Outport  Port=4  VectorParamsAs1DForOutWhenUnconnected=off
  wires:
  BusCreator1/1 -> Terminator/1  "Aero IF (in)"
  Demux2/13 -> BusCreator2/9  "car Aero Trq_1 z"
  Demux2/12 -> BusCreator2/8  "car Aero Trq_1 y"
  Demux2/11 -> BusCreator2/7  "car Aero Trq_1 x"
  Demux2/10 -> BusCreator2/6  "car Aero Frc_1 z"
  Demux2/9 -> BusCreator2/5  "car Aero Frc_1 y"
  Demux2/8 -> BusCreator2/4  "car Aero Frc_1 x"
  Demux2/7 -> BusCreator2/3  "car Aero PoA_1 z"
  Demux2/6 -> BusCreator2/2  "car Aero PoA_1 y"
  Demux2/5 -> BusCreator2/1  "car Aero PoA_1 x"
  Demux2/4 -> BusCreator1/4  "car Aero tau_1"
  Demux2/3 -> BusCreator1/3  "car Aero ApproachVel_1 z"
  Demux2/2 -> BusCreator1/2  "car Aero ApproachVel_1 y"
  Demux2/1 -> BusCreator1/1  "car Aero ApproachVel_1 x"
  Demux/16 -> Bus Creator8/16  "Car Load_3 tz"
  Demux/15 -> Bus Creator8/15  "Car Load_3 ty"
  Demux/14 -> Bus Creator8/14  "Car Load_3 tx"
  Demux/13 -> Bus Creator8/13  "Car Load_3 mass"
  Demux1/12 -> Bus Creator1/12  "Car Virtual Trq_0 z"
  Demux1/11 -> Bus Creator1/11  "Car Virtual Trq_0 y"
  Demux1/10 -> Bus Creator1/10  "Car Virtual Trq_0 x"
  Demux1/9 -> Bus Creator1/9  "Car Virtual Trq_1 z"
  Demux1/8 -> Bus Creator1/8  "Car Virtual Trq_1 y"
  Demux1/7 -> Bus Creator1/7  "Car Virtual Trq_1 x"
  Demux1/6 -> Bus Creator1/6  "Car Virtual Frc_0 z"
  Demux1/5 -> Bus Creator1/5  "Car Virtual Frc_0 y"
  Demux1/4 -> Bus Creator1/4  "Car Virtual Frc_0 x"
  Sync_In/1 -> Forces/1
  Forces/1 -> Sync_Out/1
  BusCreator2/1 -> Car.Aero/1
  Demux1/1 -> Bus Creator1/1  "Car Virtual Frc_1 x"
  Demux1/2 -> Bus Creator1/2  "Car Virtual Frc_1 y"
  Demux1/3 -> Bus Creator1/3  "Car Virtual Frc_1 z"
  Forces/3 -> Demux2/1
  Forces/2 -> Demux1/1
  Bus Creator1/1 -> Car.Virtual/1
  Bus Creator8/1 -> Car.Load/1
  Demux/1 -> Bus Creator8/1  "Car Load_0 mass"
  Demux/2 -> Bus Creator8/2  "Car Load_0 tx"
  Demux/3 -> Bus Creator8/3  "Car Load_0 ty"
  Demux/4 -> Bus Creator8/4  "Car Load_0 tz"
  Demux/5 -> Bus Creator8/5  "Car Load_1 mass"
  Demux/6 -> Bus Creator8/6  "Car Load_1 tx"
  Demux/7 -> Bus Creator8/7  "Car Load_1 ty"
  Demux/8 -> Bus Creator8/8  "Car Load_1 tz"
  Demux/9 -> Bus Creator8/9  "Car Load_2 mass"
  Demux/10 -> Bus Creator8/10  "Car Load_2 tx"
  Demux/11 -> Bus Creator8/11  "Car Load_2 ty"
  Demux/12 -> Bus Creator8/12  "Car Load_2 tz"
  Forces/4 -> Demux/1
